simulink model "sldvmiscovtool_sample_fixpt"  (Simulink 7.3)
settings: Solver=FixedStepDiscrete  StartTime=0.0  StopTime=50  FixedStep=0.01  RelTol=1e-3
undefined symbols (not defined in the file or in its folder): DiscIntNeverNeededParam
Description:
  | Cruise Control Test Generation Example
settings Model: Creator=The MathWorks Inc.  LastModifiedBy=itoy  CovMetricSettings=dcme  CovHtmlReporting=off  covSaveCumulativeToWorkspaceVar=off  CovSaveSingleToWorkspaceVar=off  ExtModeAutoUpdateStatusClock=off
settings DataIOCC: LimitDataPoints=off  SaveFormat=StructureWithTime  SaveOutput=off  SignalLogging=off  SaveTime=off
settings OptimizationCC: InlineParams=on  InlineInvariantSignals=on  InitFltsAndDblsToZero=on
settings DebuggingCC: SaveWithParameterizedLinksMsg=none  SignalResolutionControl=TryResolveAllWithWarning  ParameterDowncastMsg=warning  ParameterOverflowMsg=warning
settings HardwareCC: TargetHWDeviceType=32-bit Generic
settings GRTTargetCC: TargetFcnLib=ansi_tfl_tmw.mat
settings ConfigComp: Description=Design Verifier Custom Configuration Component  DVMaxProcessTime=1  DVDisplayUnsatisfiableObjectives=on  DVAutomaticStubbing=off  DVMakeOutputFilesUnique=off  DVModelCoverageObjectives=MCDC  DVMaxTestCaseSteps=500  DVTestSuiteOptimization=CombinedObjectives  DVAssertions=EnableAll  DVProofAssumptions=EnableAll  DVProvingStrategy=FindViolation  DVSaveHarnessModel=on  DVSaveReport=on  DVDisplayReport=off

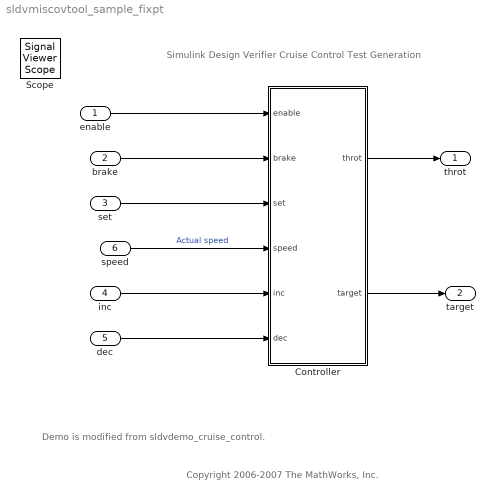
== system sldvmiscovtool_sample_fixpt ==
  note: Simulink Design Verifier
      | Cruise Control Test Generation
  note: Copyright 2006-2007 The MathWorks, Inc.
  note: Demo is modified from sldvdemo_cruise_control.
  enable : Inport  DataType=boolean  OutDataType=sfix(16)  OutScaling=2^0  OutDataTypeStr=boolean  Interpolate=off
  brake : Inport  Port=2  DataType=boolean  OutDataType=sfix(16)  OutScaling=2^0  OutDataTypeStr=boolean  Interpolate=off
  set : Inport  Port=3  DataType=boolean  OutDataType=sfix(16)  OutScaling=2^0  OutDataTypeStr=boolean  Interpolate=off
  inc : Inport  Port=4  DataType=boolean  OutDataType=sfix(16)  OutScaling=2^0  OutDataTypeStr=boolean  Interpolate=off
  dec : Inport  Port=5  DataType=boolean  OutDataType=sfix(16)  OutScaling=2^0  OutDataTypeStr=boolean  Interpolate=off
  speed : Inport  Port=6  DataType=Specify via dialog  OutDataType=fixdt(1,16,8)  OutDataTypeStr=fixdt(1,16,8)  Interpolate=off
  Controller : Subsystem
  throt : Outport  OutDataType=sfix(16)  OutScaling=2^0
  target : Outport  Port=2  OutDataType=sfix(16)  OutScaling=2^0
  Scope : SignalViewerScope  IOType=viewer  RefreshTime=0.035000
  wires:
  enable/1 -> Controller/1(enable)
  brake/1 -> Controller/2(brake)
  set/1 -> Controller/3(set)
  Controller/1(throt) -> throt/1
  inc/1 -> Controller/5(inc)
  dec/1 -> Controller/6(dec)
  Controller/2(target) -> target/1
  speed/1 -> Controller/4(speed)  "Actual speed"

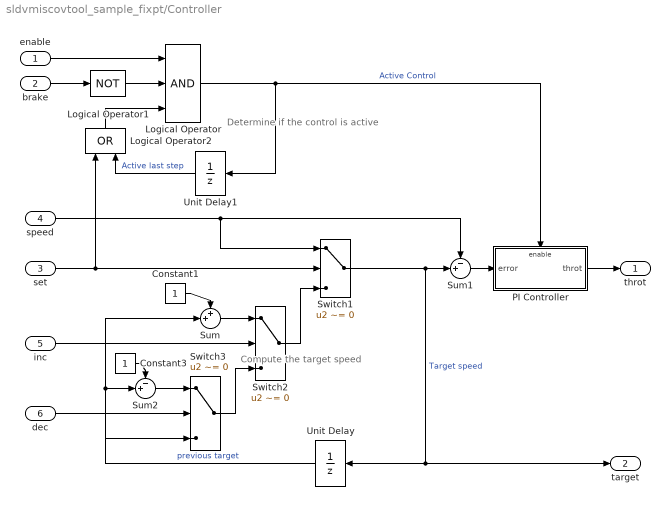
== system sldvmiscovtool_sample_fixpt/Controller ==
  note: Determine if the
      | control is active
  note: Compute the
      | target speed
  enable : Inport  DataType=boolean  OutDataType=sfix(16)  OutScaling=2^0  OutDataTypeStr=boolean
  brake : Inport  Port=2  DataType=boolean  OutDataType=sfix(16)  OutScaling=2^0  OutDataTypeStr=boolean
  set : Inport  Port=3  DataType=boolean  OutDataType=sfix(16)  OutScaling=2^0  OutDataTypeStr=boolean
  speed : Inport  Port=4  DataType=Specify via dialog  OutDataType=fixdt(1,16,8)  OutDataTypeStr=fixdt(1,16,8)
  inc : Inport  Port=5  DataType=boolean  OutDataType=sfix(16)  OutScaling=2^0  OutDataTypeStr=boolean
  dec : Inport  Port=6  DataType=boolean  OutDataType=fixdt(1,16,8)  OutScaling=2^0  OutDataTypeStr=boolean
  Constant1 : Constant  OutDataType=sfix(16)  OutScaling=2^0  OutDataTypeStr=Inherit: Inherit via back propagation
  Constant3 : Constant  OutDataType=sfix(16)  OutScaling=2^0  OutDataTypeStr=Inherit: Inherit via back propagation
  Logical Operator : Logic  Inputs=3  AllPortsSameDT=off  OutDataTypeMode=boolean  OutDataTypeStr=boolean
  Logical Operator1 : Logic  Operator=NOT  AllPortsSameDT=off  OutDataTypeMode=boolean  OutDataTypeStr=boolean
  Logical Operator2 : Logic  Operator=OR  AllPortsSameDT=off  OutDataTypeMode=boolean  OutDataTypeStr=boolean
  PI Controller : Subsystem
  Sum : Sum  Inputs=++|  OutDataType=sfix(16)  OutScaling=2^0
  Sum1 : Sum  Inputs=-+|  OutDataType=sfix(16)  OutScaling=2^0
  Sum2 : Sum  Inputs=-+|  OutDataType=sfix(16)  OutScaling=2^0
  Switch1 : Switch  Criteria=u2 ~= 0
  Switch2 : Switch  Criteria=u2 ~= 0
  Switch3 : Switch  Criteria=u2 ~= 0
  Unit Delay : UnitDelay  SampleTime=0.01
  Unit Delay1 : UnitDelay  SampleTime=0.01
  throt : Outport  OutDataType=sfix(16)  OutScaling=2^0
  target : Outport  Port=2  OutDataType=sfix(16)  OutScaling=2^0
  wires:
  brake/1 -> Logical Operator1/1
  enable/1 -> Logical Operator/1
  Logical Operator1/1 -> Logical Operator/2
  set/1 -> Switch1/2, Logical Operator2/1
  speed/1 -> Sum1/1, Switch1/1
  inc/1 -> Switch2/2
  Constant1/1 -> Sum/1
  Sum/1 -> Switch2/1
  dec/1 -> Switch3/2
  Constant3/1 -> Sum2/1
  Sum2/1 -> Switch3/1
  Switch2/1 -> Switch1/3
  Switch3/1 -> Switch2/3
  Unit Delay/1 -> Sum/2, Sum2/2, Switch3/3  "previous target"
  Switch1/1 -> Unit Delay/1, target/1, Sum1/2  "Target speed"
  Logical Operator2/1 -> Logical Operator/3
  Unit Delay1/1 -> Logical Operator2/2  "Active last step"
  Logical Operator/1 -> Unit Delay1/1, PI Controller/Enable  "Active Control"
  Sum1/1 -> PI Controller/1(error)
  PI Controller/1(throt) -> throt/1

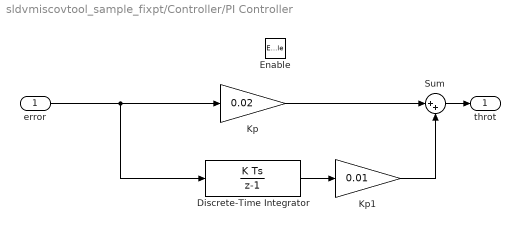
== system sldvmiscovtool_sample_fixpt/Controller/PI Controller ==
  error : Inport  OutDataType=sfix(16)  OutScaling=2^0
  Enable : EnablePort
  Discrete-Time Integrator : DiscreteIntegrator  SampleTime=0.01  OutDataTypeMode=Specify via dialog  OutDataType=fixdt(1,16,8)  OutDataTypeStr=fixdt(1,16,8)  LimitOutput=on  UpperSaturationLimit=15  LowerSaturationLimit=-5  ICPrevOutput=DiscIntNeverNeededParam  ICPrevScaledInput=DiscIntNeverNeededParam
  Kp : Gain  Gain=0.02  ParameterDataType=sfix(16)  ParameterScaling=2^0  OutDataType=sfix(16)  OutScaling=2^0  OutDataTypeStr=Inherit: Same as input
  Kp1 : Gain  Gain=0.01  ParameterDataType=sfix(16)  ParameterScaling=2^0  OutDataType=sfix(16)  OutScaling=2^0  OutDataTypeStr=Inherit: Same as input  ParamDataTypeStr=Inherit: Same as input
  Sum : Sum  Inputs=|++  OutDataType=sfix(16)  OutScaling=2^0
  throt : Outport  OutDataType=sfix(16)  OutScaling=2^0
  wires:
  Kp/1 -> Sum/1
  Kp1/1 -> Sum/2
  Discrete-Time Integrator/1 -> Kp1/1
  error/1 -> Kp/1, Discrete-Time Integrator/1
  Sum/1 -> throt/1
